simulink model "lab_07_01"  (R2024b)
settings: Solver=VariableStepAuto  StartTime=0.0  StopTime=10.0  RelTol=1e-3
undefined symbols (not defined in the file or in its folder): dspblkCoreblockFVToolHelper, gcbh
libraries: commanapbnd3 x2
settings Model: LastModifiedBy=LENOVO

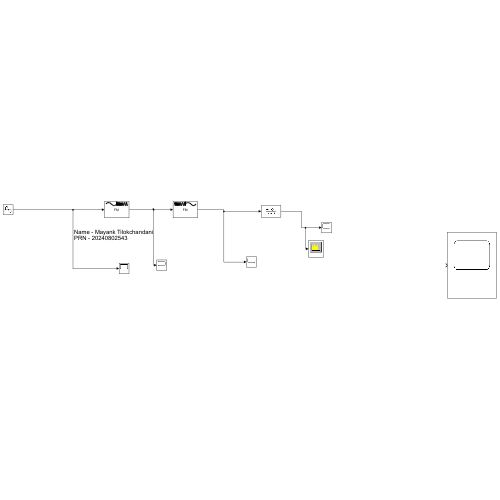
[thumbnail: Simulink's stored preview of the top-level diagram]
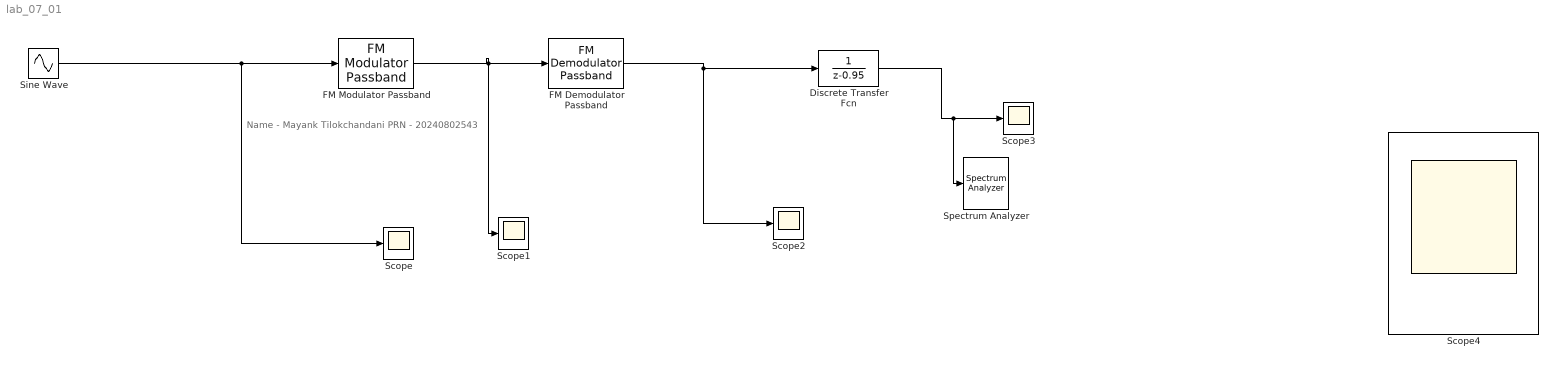
== system lab_07_01 ==
  note: Name - Mayank Tilokchandani
      | PRN - 20240802543
  Discrete Transfer Fcn : DiscreteTransferFcn  LoadFcn=dspblkCoreblockFVToolHelper(gcbh,'load');  Denominator=[1 -0.95]
      settings: CopyFcn=dspblkCoreblockFVToolHelper(gcbh,'copy');  DeleteFcn=dspblkCoreblockFVToolHelper(gcbh,'close');  ModelCloseFcn=dspblkCoreblockFVToolHelper(gcbh,'close');  PreSaveFcn=dspblkCoreblockFVToolHelper(gcbh,'presave');  PostSaveFcn=dspblkCoreblockFVToolHelper(gcbh,'postsave');  CloseFcn=dspblkCoreblockFVToolHelper(gcbh,'close');
  FM Demodulator Passband : commanapbnd3/FM Demodulator Passband  Fc=100  Ph=pi/2  Kc=10  Ho=100
  FM Modulator Passband : commanapbnd3/FM Modulator Passband  Fc=100  Ph=0  Kc=10
  Scope{,1..4} (5 alike) : Scope
  Sine Wave : Sin  Amplitude=5  Frequency=2*pi*0.9  SampleTime=0.001
  Spectrum Analyzer : SpectrumAnalyzer  WindowPosition=[477.000000,207.000000,800.000000,500.000000,]  Visible=on  ScopeFrameLocation=window  SampleRate=44.1e3  PlotAsTwoSidedSpectrum=off  FrequencyScale=Log  WindowInvariantSamplesPerUpdate=on  FrequencySpan=Start and stop frequencies  StartFrequency=0  StopFrequency=500  YLimits=[22.76563058119075,52.430386225196884]
  wires:
  Sine Wave/1 -> Scope/1, FM Modulator Passband/1
  FM Modulator Passband/1 -> FM Demodulator Passband/1, Scope1/1
  FM Demodulator Passband/1 -> Discrete Transfer Fcn/1, Scope2/1
  Discrete Transfer Fcn/1 -> Spectrum Analyzer/1, Scope3/1
